simulink model "Mini_projet"  (R2017a)
settings: Solver=VariableStepAuto  StartTime=0.0  StopTime=10  RelTol=1e-3
values from neighbouring files (symbols this model uses):
  b = 2    [Adaptive_Control_Linear.m]    (also in Adaptive_control_Non_linear.m; HOSM.m = 1; feedback-integrator.m = 3; mini_projet.m = 3)
  k1 = 143/(1+b)    (= 35.75)    [feedback-integrator.m]    (also in mini_projet.m; projet_AAV.m = 1)
  k2 = 23/(1+b)    (= 5.75)    [feedback-integrator.m]    (also in mini_projet.m; projet_AAV.m = 1)
settings Model: Creator=firass2019  LastModifiedBy=firass2019

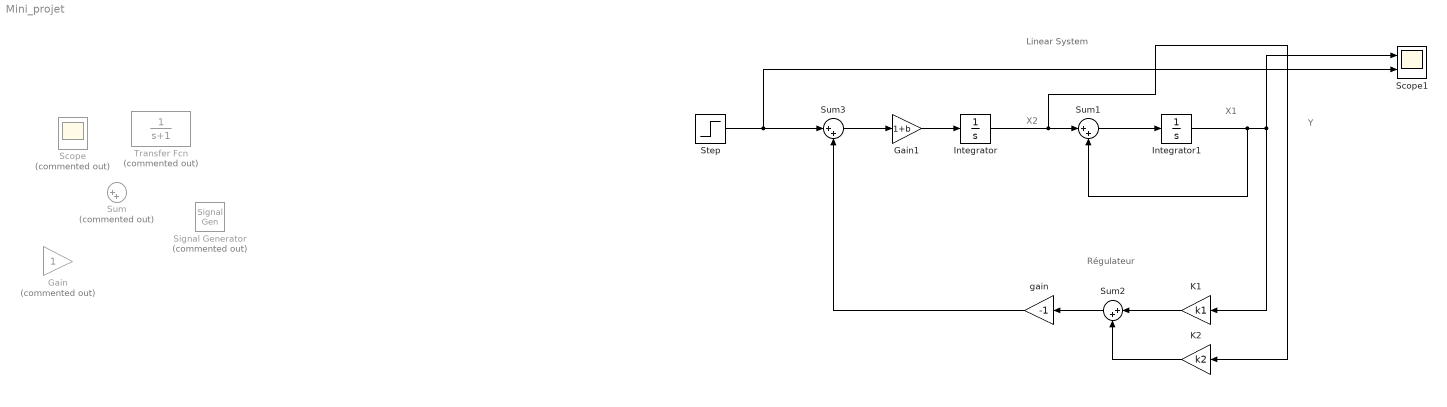
== system Mini_projet ==
  note: Régulateur
  note: Y
  note: X1
  note: X2
  note: Linear System
  Gain : Gain  Commented=on
  Gain1 : Gain  Gain=1+b
  Integrator : Integrator  InitialCondition=0.1
  Integrator1 : Integrator  InitialCondition=0.1
  K1 : Gain  Gain=k1
  K2 : Gain  Gain=k2
  Scope : Scope  Commented=on
  Scope1 : Scope  NumInputPorts=2
  Signal Generator : SignalGenerator  Commented=on  Units=rad/sec
  Step : Step  SampleTime=0
  Sum : Sum  Commented=on  Inputs=|++
  Sum1 : Sum  Inputs=|++
  Sum2 : Sum  Inputs=|++
  Sum3 : Sum  Inputs=|++
  Transfer Fcn : TransferFcn  Commented=on  Denominator=[1 1]
  gain : Gain  Gain=-1
  wires:
  Sum1/1 -> Integrator1/1
  Integrator1/1 -> Scope1/1, K1/1, Sum1/2
  K1/1 -> Sum2/1
  K2/1 -> Sum2/2
  Sum2/1 -> gain/1
  Gain1/1 -> Integrator/1
  gain/1 -> Sum3/2
  Sum3/1 -> Gain1/1
  Integrator/1 -> K2/1, Sum1/1
  Step/1 -> Scope1/2, Sum3/1
